simulink model "slGTC_3gdl"  (Simulink 9.0)
settings: Solver=ode45  StartTime=0.0  StopTime=Tsim  MaxStep=1e-3  RelTol=1e-8  EnableMultiTasking=on
values from neighbouring files (symbols this model uses):
  XYZfin = [in(4) in(5) in(6)]'    [GTCL_R3GDL.m]    (also in main.m = CinematicaDirecta([1 1 1]); simular.m = CinematicaDirecta([1 1 1]))
  XYZini = CinematicaDirecta([0 0 0])    [main.m]    (also in simular.m)
undefined symbols (not defined in the file or in its folder): Duracion, kd1, kd2, kd3, ki1, ki2, ki3, kp1, kp2, kp3, N_puntos, Tini
settings Model: Creator=Manuel G. Ortega  LastModifiedBy=Alvaro  ExtModeTrigMode=oneshot  ExtModeArmWhenConnect=off
settings DataIOCC: SignalLoggingSaveFormat=ModelDataLogs
settings OptimizationCC: BooleanDataType=off  ExpressionDepthLimit=2147483647  InitFltsAndDblsToZero=on
settings DebuggingCC: SaveWithParameterizedLinksMsg=none  SignalResolutionControl=TryResolveAllWithWarning  MultiTaskDSMMsg=warning  MultiTaskCondExecSysMsg=none  FcnCallInpInsideContextMsg=warning  StateNameClashWarn=warning  StrictBusMsg=None
settings HardwareCC: TargetUnknown=on
settings GRTTargetCC: TargetFcnLib=ansi_tfl_tmw.mat  GeneratePreprocessorConditionals=Disable all  CombineOutputUpdateFcns=off  GRTInterface=on
settings ConfigComp: CovSFcnEnable=off

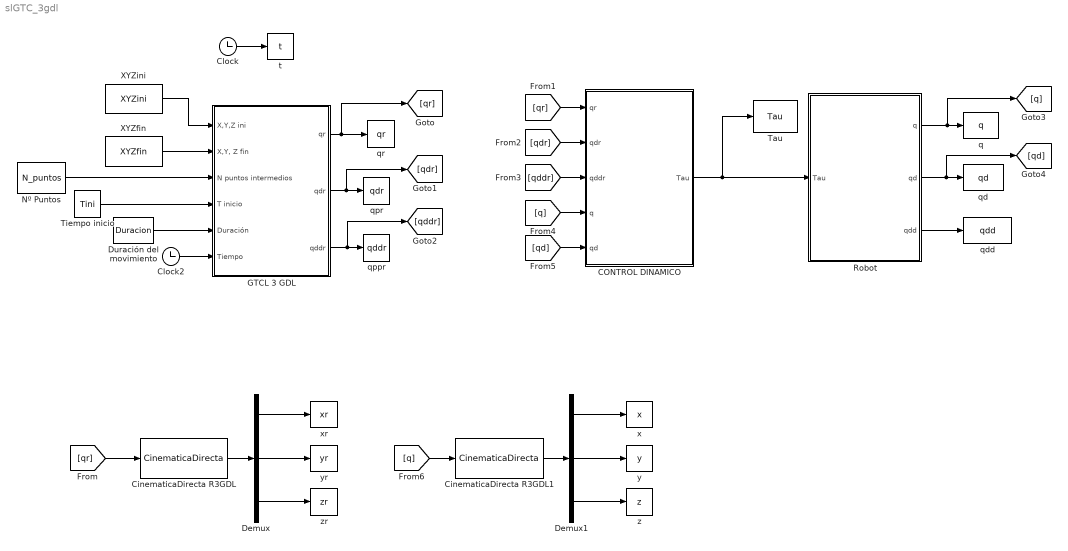
== system slGTC_3gdl ==
  CONTROL DINAMICO : Subsystem
  CinematicaDirecta R3GDL : MATLABFcn  MATLABFcn=CinematicaDirecta
  CinematicaDirecta R3GDL1 : MATLABFcn  MATLABFcn=CinematicaDirecta
  Clock : Clock
  Clock2 : Clock
  Demux : Demux  Outputs=3
  Demux1 : Demux  Outputs=3
  Duración del movimiento : Constant  Value=Duracion
  GTCL 3 GDL : Subsystem
  Nº Puntos : Constant  Value=N_puntos
  Robot : Subsystem
  "Tau " : ToWorkspace  VariableName=Tau  SampleTime=-1
  Tiempo inicio : Constant  Value=Tini
  XYZfin : Constant  Value=XYZfin
  XYZini : Constant  Value=XYZini
  q : ToWorkspace  VariableName=q  SampleTime=-1
  qd : ToWorkspace  VariableName=qd  SampleTime=-1
  qdd : ToWorkspace  VariableName=qdd  SampleTime=-1
  qppr : ToWorkspace  VariableName=qddr  SampleTime=-1
  qpr : ToWorkspace  VariableName=qdr  SampleTime=-1
  qr : ToWorkspace  VariableName=qr  SampleTime=-1
  t : ToWorkspace  VariableName=t  SampleTime=-1
  x : ToWorkspace  VariableName=x  SampleTime=-1
  xr : ToWorkspace  VariableName=xr  SampleTime=-1
  y : ToWorkspace  VariableName=y  SampleTime=-1
  yr : ToWorkspace  VariableName=yr  SampleTime=-1
  z : ToWorkspace  VariableName=z  SampleTime=-1
  zr : ToWorkspace  VariableName=zr  SampleTime=-1
  wires:
  Clock/1 -> t/1
  Clock2/1 -> GTCL 3 GDL/6(Tiempo)
  Duración del movimiento/1 -> GTCL 3 GDL/5(Duración)
  Tiempo inicio/1 -> GTCL 3 GDL/4(T inicio)
  Nº Puntos/1 -> GTCL 3 GDL/3(N puntos intermedios)
  XYZfin/1 -> GTCL 3 GDL/2("X,Y, Z fin")
  XYZini/1 -> GTCL 3 GDL/1(X,Y,Z ini)
  GTCL 3 GDL/1(qr) -> [qr], qr/1
  GTCL 3 GDL/2(qdr) -> [qdr], qpr/1
  GTCL 3 GDL/3(qddr) -> [qddr], qppr/1
  [qr] -> CinematicaDirecta R3GDL/1
  CinematicaDirecta R3GDL/1 -> Demux/1
  Demux/1 -> xr/1
  Demux/2 -> yr/1
  Demux/3 -> zr/1
  CONTROL DINAMICO/1(Tau) -> "Tau "/1, Robot/1(Tau)
  Robot/3(qdd) -> qdd/1
  Robot/2(qd) -> [qd], qd/1
  Robot/1(q) -> [q], q/1
  [qr] -> CONTROL DINAMICO/1(qr)
  [qdr] -> CONTROL DINAMICO/2(qdr)
  [qddr] -> CONTROL DINAMICO/3(qddr)
  [q] -> CONTROL DINAMICO/4(q)
  [qd] -> CONTROL DINAMICO/5(qd)
  Demux1/3 -> z/1
  Demux1/2 -> y/1
  Demux1/1 -> x/1
  CinematicaDirecta R3GDL1/1 -> Demux1/1
  [q] -> CinematicaDirecta R3GDL1/1

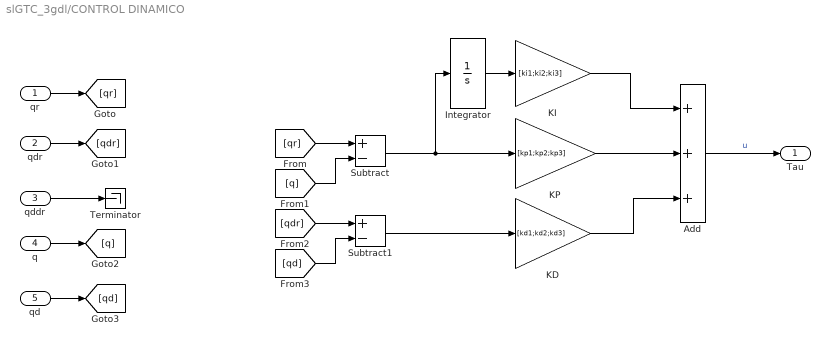
== system slGTC_3gdl/CONTROL DINAMICO ==
  qr : Inport
  qdr : Inport  Port=2
  qddr : Inport  Port=3
  q : Inport  Port=4
  qd : Inport  Port=5
  Add : Sum  Inputs=+++
  Integrator : Integrator
  KD : Gain  Gain=[kd1;kd2;kd3]
  KI : Gain  Gain=[ki1;ki2;ki3]
  KP : Gain  Gain=[kp1;kp2;kp3]
  Subtract : Sum  Inputs=+-
  Subtract1 : Sum  Inputs=+-
  Terminator : Terminator
  Tau : Outport
  wires:
  qr/1 -> [qr]
  qdr/1 -> [qdr]
  qddr/1 -> Terminator/1
  q/1 -> [q]
  qd/1 -> [qd]
  [qr] -> Subtract/1
  [q] -> Subtract/2
  [qdr] -> Subtract1/1
  [qd] -> Subtract1/2
  Add/1 -> Tau/1  "u"
  Integrator/1 -> KI/1
  KP/1 -> Add/2
  KD/1 -> Add/3
  KI/1 -> Add/1
  Subtract1/1 -> KD/1
  Subtract/1 -> Integrator/1, KP/1

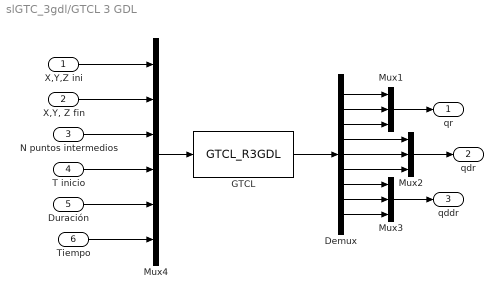
== system slGTC_3gdl/GTCL 3 GDL ==
  X,Y,Z ini : Inport
  "X,Y, Z fin" : Inport  Port=2
  N puntos intermedios : Inport  Port=3
  T inicio : Inport  Port=4
  Duración : Inport  Port=5
  Tiempo : Inport  Port=6
  Demux : Demux  Outputs=9
  GTCL : MATLABFcn  MATLABFcn=GTCL_R3GDL  OutputDimensions=9
  Mux1 : Mux  Inputs=3
  Mux2 : Mux  Inputs=3
  Mux3 : Mux  Inputs=3
  Mux4 : Mux  Inputs=6
  qr : Outport
  qdr : Outport  Port=2
  qddr : Outport  Port=3
  wires:
  Mux1/1 -> qr/1
  Mux4/1 -> GTCL/1
  X,Y,Z ini/1 -> Mux4/1
  "X,Y, Z fin"/1 -> Mux4/2
  N puntos intermedios/1 -> Mux4/3
  T inicio/1 -> Mux4/4
  Duración/1 -> Mux4/5
  Tiempo/1 -> Mux4/6
  GTCL/1 -> Demux/1
  Demux/1 -> Mux1/1
  Demux/2 -> Mux1/2
  Demux/3 -> Mux1/3
  Mux2/1 -> qdr/1
  Demux/4 -> Mux2/1
  Demux/5 -> Mux2/2
  Demux/6 -> Mux2/3
  Mux3/1 -> qddr/1
  Demux/7 -> Mux3/1
  Demux/8 -> Mux3/2
  Demux/9 -> Mux3/3

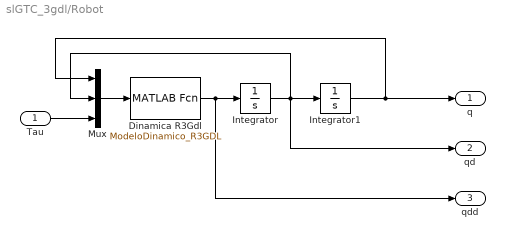
== system slGTC_3gdl/Robot ==
  Tau : Inport
  Dinamica R3Gdl : MATLABFcn  MATLABFcn=ModeloDinamico_R3GDL
  Integrator : Integrator  InitialCondition=[0;0;0];
  Integrator1 : Integrator  InitialCondition=[0;0;0]
  Mux : Mux  Inputs=3
  q : Outport
  qd : Outport  Port=2
  qdd : Outport  Port=3
  wires:
  Tau/1 -> Mux/3
  Integrator1/1 -> Mux/1, q/1
  Integrator/1 -> Mux/2, qd/1, Integrator1/1
  Dinamica R3Gdl/1 -> qdd/1, Integrator/1
  Mux/1 -> Dinamica R3Gdl/1
